simulink model "ABS_opt"  (R2017b)
settings: Solver=VariableStepAuto  StartTime=0.0  StopTime=60.0  RelTol=1e-3
InitFcn:
  | J = 1.13;
  | g = 9.81;
  | T_B = 0.1;
values from neighbouring files (symbols this model uses):
  ce = road_coeff(sel,:)    [ABS_ga.m]    (also in ABS_pso.m)
  Kpid = actSelGen(i,:)    [ABS_ga.m]    (also in ABS_pso.m = Swarm.Particles(k).X)
  lam_d = 0.2    [ABS_ga.m]    (also in ABS_pso.m)
undefined symbols (not defined in the file or in its folder): m, R, type, v_x
libraries: simulink x2
settings Model: Creator=hadlaczkyb  LastModifiedBy=hadlaczkyb

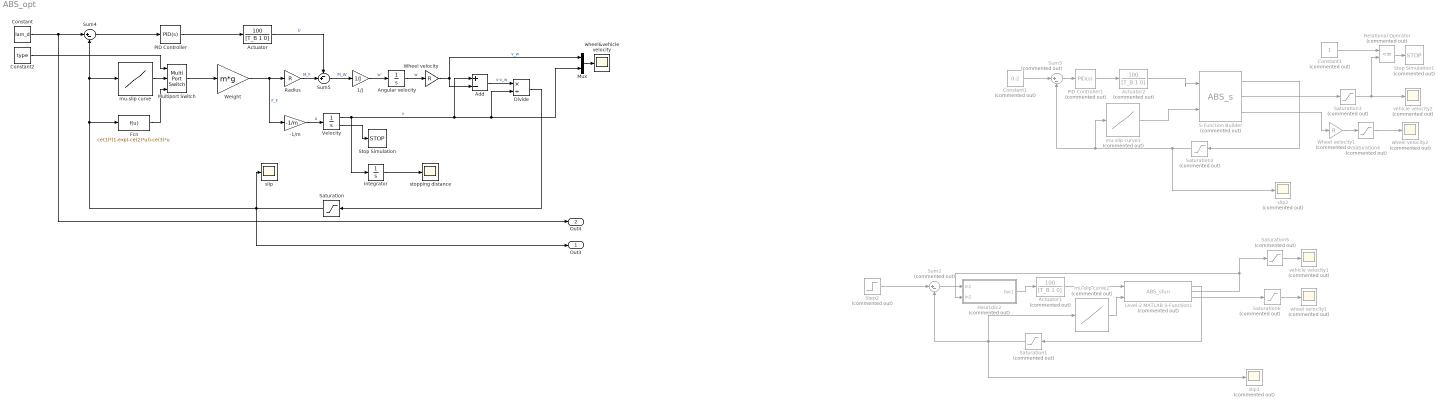
== system ABS_opt ==
  -1/m : Gain  Gain=-1/m
  1/J : Gain  Gain=1/J
  Actuator : TransferFcn  Numerator=[100]  Denominator=[T_B 1 0]
  Actuator1 : TransferFcn  Commented=on  Numerator=[0 0 100]  Denominator=[T_B 1 0]
  Actuator2 : TransferFcn  Commented=on  Numerator=[0 0 100]  Denominator=[T_B 1 0]
  Add : Sum  Inputs=+-
  Angular velocity : Integrator  InitialCondition=v_x/R  LimitOutput=on  UpperSaturationLimit=1000  LowerSaturationLimit=0
  Constant : Constant  Value=lam_d
  Constant1 : Constant  Commented=on  Value=0.2
  Constant2 : Constant  Value=type
  Constant3 : Constant  Commented=on
  Divide : Product  Inputs=*/
  Fcn : Fcn  Expr=ce(1)*(1-exp(-ce(2)*u))-ce(3)*u
  Heuristic2 : Subsystem  Commented=on
  Integrator : Integrator
  Level-2 MATLAB S-Function1 : M-S-Function  Commented=on  FunctionName=ABS_sfun  Parameters=27.78, 84.18, 0
  Multiport Switch : MultiPortSwitch  Inputs=2
  Mux : Mux  Inputs=2
  PID Controller : simulink/Continuous/PID Controller  Controller=PID  TimeDomain=Continuous-time  SampleTime=-1  IntegratorMethod=Forward Euler  FilterMethod=Forward Euler  Form=Parallel  UseFilter=on  ControllerParametersSource=internal  P=Kpid(1)  I=Kpid(2)  D=Kpid(3)  N=1000  InitialConditionSource=internal  InitialConditionForIntegrator=0  InitialConditionForFilter=0  ExternalReset=none  LimitOutput=off  UpperSaturationLimit=inf  LowerSaturationLimit=-inf  LinearizeAsGain=on  AntiWindupMode=none  Kb=1  TrackingMode=off  Kt=1  PParamMin=[]  PParamMax=[]  IParamMin=[]  IParamMax=[]  DParamMin=[]  DParamMax=[]  NParamMin=[]  NParamMax=[]  KbParamMin=[]  KbParamMax=[]  KtParamMin=[]  KtParamMax=[]  POutMin=[]  POutMax=[]  IOutMin=[]  IOutMax=[]  DOutMin=[]  DOutMax=[]  NOutMin=[]  NOutMax=[]  KbOutMin=[]  KbOutMax=[]  KtOutMin=[]  KtOutMax=[]  IntegratorOutMin=[]  IntegratorOutMax=[]  FilterOutMin=[]  FilterOutMax=[]  SumOutMin=[]  SumOutMax=[]  SumI1OutMin=[]  SumI1OutMax=[]  SumI2OutMin=[]  SumI2OutMax=[]  SumI3OutMin=[]  SumI3OutMax=[]  SumDOutMin=[]  SumDOutMax=[]  SaturationOutMin=[]  SaturationOutMax=[]  IntegratorContinuousStateAttributes=''  IntegratorStateMustResolveToSignalObject=off  IntegratorRTWStateStorageClass=Auto  FilterContinuousStateAttributes=''  FilterStateMustResolveToSignalObject=off  FilterRTWStateStorageClass=Auto  DifferentiatorICPrevScaledInput=0  DifferentiatorOutMin=[]  DifferentiatorOutMax=[]  InitialConditionSetting=State (most efficient)  FilterDiffOutCoefMin=[]  FilterDiffOutCoefMax=[]  SumDenOutMin=[]  SumDenOutMax=[]  SumNumOutMin=[]  SumNumOutMax=[]  ReciprocalOutMin=[]  ReciprocalOutMax=[]  DivideOutMin=[]  DivideOutMax=[]  TunerSelectOption=Transfer Function Based (PID Tuner App)
  PID Controller1 : simulink/Continuous/PID Controller  Commented=on  Controller=PID  TimeDomain=Continuous-time  SampleTime=-1  IntegratorMethod=Forward Euler  FilterMethod=Forward Euler  Form=Parallel  UseFilter=on  ControllerParametersSource=internal  P=627.569  I=0  D=127.077  N=1000  InitialConditionSource=internal  InitialConditionForIntegrator=0  InitialConditionForFilter=0  ExternalReset=none  LimitOutput=off  UpperSaturationLimit=inf  LowerSaturationLimit=-inf  LinearizeAsGain=on  AntiWindupMode=none  Kb=1  TrackingMode=off  Kt=1  PParamMin=[]  PParamMax=[]  IParamMin=[]  IParamMax=[]  DParamMin=[]  DParamMax=[]  NParamMin=[]  NParamMax=[]  KbParamMin=[]  KbParamMax=[]  KtParamMin=[]  KtParamMax=[]  POutMin=[]  POutMax=[]  IOutMin=[]  IOutMax=[]  DOutMin=[]  DOutMax=[]  NOutMin=[]  NOutMax=[]  KbOutMin=[]  KbOutMax=[]  KtOutMin=[]  KtOutMax=[]  IntegratorOutMin=[]  IntegratorOutMax=[]  FilterOutMin=[]  FilterOutMax=[]  SumOutMin=[]  SumOutMax=[]  SumI1OutMin=[]  SumI1OutMax=[]  SumI2OutMin=[]  SumI2OutMax=[]  SumI3OutMin=[]  SumI3OutMax=[]  SumDOutMin=[]  SumDOutMax=[]  SaturationOutMin=[]  SaturationOutMax=[]  IntegratorContinuousStateAttributes=''  IntegratorStateMustResolveToSignalObject=off  IntegratorRTWStateStorageClass=Auto  FilterContinuousStateAttributes=''  FilterStateMustResolveToSignalObject=off  FilterRTWStateStorageClass=Auto  DifferentiatorICPrevScaledInput=0  DifferentiatorOutMin=[]  DifferentiatorOutMax=[]  InitialConditionSetting=State (most efficient)  FilterDiffOutCoefMin=[]  FilterDiffOutCoefMax=[]  SumDenOutMin=[]  SumDenOutMax=[]  SumNumOutMin=[]  SumNumOutMax=[]  ReciprocalOutMin=[]  ReciprocalOutMax=[]  DivideOutMin=[]  DivideOutMax=[]  TunerSelectOption=Transfer Function Based (PID Tuner App)
  Radius : Gain  Gain=R
  Relational Operator : RelationalOperator  Commented=on  Operator=<=  OutDataTypeStr=boolean  RndMeth=Simplest
  S-Function Builder : S-Function  Commented=on  InitFcn=try, set_param(gcb,'FunctionName','ABS_s'), end  FunctionName=ABS_s  Parameters=342,0.33,1.13,27.78,9.81,1.281,23.99,0.520  SFunctionModules=ABS_s_wrapper  SFunctionDeploymentMode=off  EnableBusSupport=off  mask(S-Function Builder){}
      mask help: Simulink:masks:SFunctionBuilder_MD
      mask init:
      | val = [[.9  0.75 0.75 1 1 .9 .9 1]',[1 1 0.75 0.75 .9 .9 1 .9]'];try , sys = get_param(gcb,'SfunBuilderFcnName');if isempty(sys), sys = get_param(gcb,'FunctionName'); end,catch, sys = get_param(gcb,'FunctionName'); end
      settings: CopyFcn=set_param(gcbh,'LinkStatus','none')  PreSaveFcn=try, set_param(gcb,'FunctionName','ABS_s'), end  OpenFcn=sfunctionwizard(gcbh)
      mask Display: plot(val(:,1),val(:,2)),disp(sys), port_label('input',1,'u'), port_label('input',2,'mu'), port_label('output',1,'lam'), port_label('output',2,'v_x'), port_label('output',3,'w')
  Saturation : Saturate  UpperLimit=1  LowerLimit=0
  Saturation1 : Saturate  Commented=on  UpperLimit=1  LowerLimit=0
  Saturation2 : Saturate  Commented=on  UpperLimit=1  LowerLimit=0
  Saturation{3..6} (4 alike) : Saturate  Commented=on  UpperLimit=inf  LowerLimit=0
  Step2 : Step  Commented=on  After=0.2  SampleTime=0
  Stop Simulation : Stop
  Stop Simulation1 : Stop  Commented=on
  Sum2 : Sum  Commented=on  Inputs=|+-
  Sum3 : Sum  Commented=on  Inputs=|+-
  Sum4 : Sum  Inputs=|+-
  Sum5 : Sum  Inputs=-+|
  Velocity : Integrator  InitialCondition=v_x  LimitOutput=on  UpperSaturationLimit=1000  LowerSaturationLimit=1  ShowSaturationPort=on
  Weight : Gain  Gain=m*g
  Wheel velocity : Gain  Gain=R
  Wheel velocity1 : Gain  Commented=on  Gain=R
  mu-slip curve : Lookup_n-D  NumberOfTableDimensions=1  BreakpointsSpecification=Even spacing  BreakpointsForDimension1=[-5:5]  BreakpointsForDimension1FirstPoint=0  BreakpointsForDimension1Spacing=0.05  Table=[0,0.4,0.8,0.97,1,0.98,0.96,0.94,0.92,0.9,0.88,0.855,0.83,0.81,0.79,0.77,0.75,0.73,0.72,0.71,0.7]  InternalRulePriority=Speed  RndMeth=Simplest  InputSameDT=on
  mu-slip curve1 : Lookup_n-D  Commented=on  NumberOfTableDimensions=1  BreakpointsSpecification=Even spacing  BreakpointsForDimension1=[-5:5]  BreakpointsForDimension1FirstPoint=0  BreakpointsForDimension1Spacing=0.05  Table=[0,0.4,0.8,0.97,1,0.98,0.96,0.94,0.92,0.9,0.88,0.855,0.83,0.81,0.79,0.77,0.75,0.73,0.72,0.71,0.7]  InternalRulePriority=Speed  RndMeth=Simplest  InputSameDT=on
  mu-slip curve2 : Lookup_n-D  Commented=on  NumberOfTableDimensions=1  BreakpointsSpecification=Even spacing  BreakpointsForDimension1=[-5:5]  BreakpointsForDimension1FirstPoint=0  BreakpointsForDimension1Spacing=0.05  Table=[0,0.4,0.8,0.97,1,0.98,0.96,0.94,0.92,0.9,0.88,0.855,0.83,0.81,0.79,0.77,0.75,0.73,0.72,0.71,0.7]  InternalRulePriority=Speed  RndMeth=Simplest  InputSameDT=on
  slip : Scope
  slip1 : Scope  Commented=on
  slip2 : Scope  Commented=on
  stopping distance : Scope
  vehicle velocity1 : Scope  Commented=on
  vehicle velocity2 : Scope  Commented=on
  wheel velocity1 : Scope  Commented=on
  wheel velocity2 : Scope  Commented=on
  wheel&vehicle velocity : Scope
  Out3 : Outport
  Out4 : Outport  Port=2
  wires:
  Sum5/1 -> 1/J/1  "M_W"
  Add/1 -> Divide/1  "v-v_w"
  -1/m/1 -> Velocity/1  "a"
  Velocity/1 -> Add/1, Mux/2, Divide/2, Integrator/1  "v"
  Weight/1 -> Radius/1, -1/m/1  "F_F"
  Actuator/1 -> Sum5/1  "U"
  Integrator/1 -> stopping distance/1
  PID Controller/1 -> Actuator/1
  Sum4/1 -> PID Controller/1
  Angular velocity/1 -> Wheel velocity/1  "w"
  1/J/1 -> Angular velocity/1  "w'"
  Radius/1 -> Sum5/2  "M_F"
  Velocity/2 -> Stop Simulation/1
  Wheel velocity/1 -> Mux/1, Add/2  "v_w"
  Saturation4/1 -> wheel velocity2/1
  Wheel velocity1/1 -> Saturation4/1
  Level-2 MATLAB S-Function1/1 -> Saturation1/1
  mu-slip curve2/1 -> Level-2 MATLAB S-Function1/2
  Step2/1 -> Sum2/1
  Level-2 MATLAB S-Function1/2 -> Heuristic2/2(In2), Saturation5/1
  Sum3/1 -> PID Controller1/1
  Actuator2/1 -> S-Function Builder/1
  S-Function Builder/2 -> Saturation3/1
  Constant1/1 -> Sum3/1
  Saturation5/1 -> vehicle velocity1/1
  S-Function Builder/1 -> Saturation2/1
  Saturation3/1 -> Relational Operator/2, vehicle velocity2/1
  Level-2 MATLAB S-Function1/3 -> Saturation6/1
  Actuator1/1 -> Level-2 MATLAB S-Function1/1
  PID Controller1/1 -> Actuator2/1
  Heuristic2/1(Out1) -> Actuator1/1
  mu-slip curve1/1 -> S-Function Builder/2
  Saturation1/1 -> Sum2/2, mu-slip curve2/1, slip1/1
  S-Function Builder/3 -> Wheel velocity1/1
  Sum2/1 -> Heuristic2/1(In1)
  Saturation2/1 -> slip2/1, mu-slip curve1/1, Sum3/2
  Saturation6/1 -> wheel velocity1/1
  Divide/1 -> Saturation/1
  Constant/1 -> Sum4/1, Out4/1
  Saturation/1 -> Out3/1, slip/1, Fcn/1, mu-slip curve/1, Sum4/2
  Multiport Switch/1 -> Weight/1
  mu-slip curve/1 -> Multiport Switch/2
  Fcn/1 -> Multiport Switch/3
  Constant2/1 -> Multiport Switch/1
  Relational Operator/1 -> Stop Simulation1/1
  Constant3/1 -> Relational Operator/1
  Mux/1 -> wheel&vehicle velocity/1

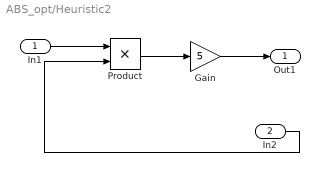
== system ABS_opt/Heuristic2 ==
  In1 : Inport
  In2 : Inport  Port=2
  Gain : Gain  Gain=5
  Product : Product
  Out1 : Outport
  wires:
  In1/1 -> Product/1
  In2/1 -> Product/2
  Product/1 -> Gain/1
  Gain/1 -> Out1/1
